simulink model "sim_cont_dig"  (R2021a)
settings: Solver=VariableStepAuto  StartTime=0.0  StopTime=5.0  RelTol=1e-3
values from neighbouring files (symbols this model uses):
  C1 = db2mag(6)*C0    [control_dig.m]
  C_dbil = (18.06 *z^2 - 29.55 *z + 12.09)/(z^2 - 1.333* z + 0.3333)    [control_dig.m]
  C_dbw = ((11.0 *z - 9.0)^2*  0.44774422771366801043768646195531)/(3.0 *z^2  - 4.0 *z + 1.0)    [control_dig.m]
  P = zpk([], [-6.96+6.55j -6.96-6.55j], Kc)    [control_dig.m]
  Ts = 20e-3    (= 0.02)    [control_dig.m]
settings Model: Creator=mathe  LastModifiedBy=mathe

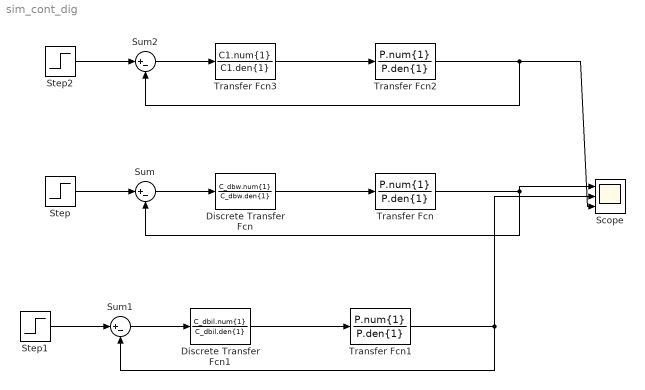
== system sim_cont_dig ==
  Discrete Transfer Fcn : DiscreteTransferFcn  Numerator=C_dbw.num{1}  Denominator=C_dbw.den{1}  SampleTime=Ts
  Discrete Transfer Fcn1 : DiscreteTransferFcn  Numerator=C_dbil.num{1}  Denominator=C_dbil.den{1}  SampleTime=Ts
  Scope : Scope  NumInputPorts=3
  Step : Step  SampleTime=0
  Step1 : Step  SampleTime=0
  Step2 : Step  SampleTime=0
  Sum : Sum  Inputs=|+-
  Sum1 : Sum  Inputs=|+-
  Sum2 : Sum  Inputs=|+-
  Transfer Fcn : TransferFcn  Numerator=P.num{1}  Denominator=P.den{1}
  Transfer Fcn1 : TransferFcn  Numerator=P.num{1}  Denominator=P.den{1}
  Transfer Fcn2 : TransferFcn  Numerator=P.num{1}  Denominator=P.den{1}
  Transfer Fcn3 : TransferFcn  Numerator=C1.num{1}  Denominator=C1.den{1}
  wires:
  Discrete Transfer Fcn/1 -> Transfer Fcn/1
  Step/1 -> Sum/1
  Transfer Fcn/1 -> Scope/1, Sum/2
  Sum/1 -> Discrete Transfer Fcn/1
  Step1/1 -> Sum1/1
  Transfer Fcn1/1 -> Scope/2, Sum1/2
  Discrete Transfer Fcn1/1 -> Transfer Fcn1/1
  Sum1/1 -> Discrete Transfer Fcn1/1
  Transfer Fcn3/1 -> Transfer Fcn2/1
  Step2/1 -> Sum2/1
  Sum2/1 -> Transfer Fcn3/1
  Transfer Fcn2/1 -> Scope/3, Sum2/2
